simulink model "uloha3simulink"  (R2019b)
settings: Solver=FixedStepAuto  StartTime=0.0  StopTime=50  FixedStep=1e-3  MaxStep=1e-4  RelTol=1e-3
values from neighbouring files (symbols this model uses):
  B = 0.1    [uloha3.m]
  b = 0.05    [uloha3.m]
  Kd = G(3)    [uloha3.m]
  Ki = G(2)    [uloha3.m]
  Kp = G(1)    [uloha3.m]
  Kv = -1/g    (= -0.101936799185)    [uloha3.m]
  l = 3    [uloha3.m]
  omega = sqrt(g/l)    [uloha3.m]
  Tm = 1    [uloha3.m]
undefined symbols (not defined in the file or in its folder): A, jerk, Kd2, Ki2, Kp2, Nel, Tvz
libraries: simulink x3, vrlib x3
settings Model: Creator=Niki  LastModifiedBy=Niki

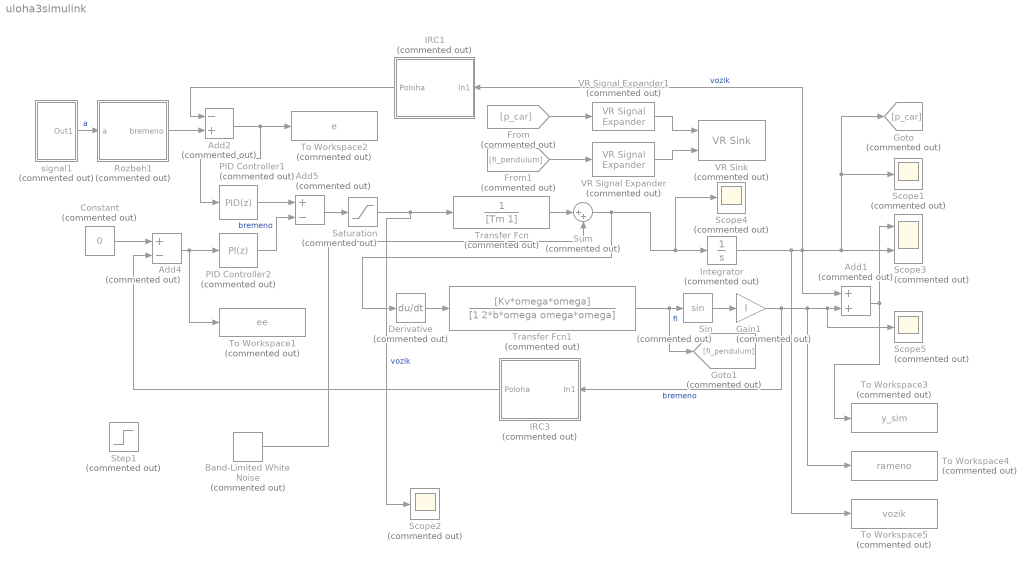
== system uloha3simulink ==
  Add1 : Sum  Commented=on
  Add2 : Sum  Commented=on  Inputs=-+
  Add4 : Sum  Commented=on  Inputs=+-
  Add5 : Sum  Commented=on  Inputs=+-
  Band-Limited White Noise : simulink/Sources/Band-Limited White Noise  Commented=on  Cov=[0.0005]  Ts=0.1  seed=[23341]
  Constant : Constant  Commented=on  Value=0
  Derivative : Derivative  Commented=on
  From : From  Commented=on  GotoTag=p_car
  From1 : From  Commented=on  GotoTag=fi_pendulum
  Gain1 : Gain  Commented=on  Gain=l
  Goto : Goto  Commented=on  GotoTag=p_car
  Goto1 : Goto  Commented=on  GotoTag=fi_pendulum
  IRC1 : Subsystem  Commented=on
  IRC3 : Subsystem  Commented=on
  Integrator : Integrator  Commented=on
  PID Controller1 : simulink/Continuous/PID Controller  Commented=on  Controller=PID  Form=Parallel  TimeDomain=Discrete-time  SampleTime=Tvz  IntegratorMethod=Forward Euler  FilterMethod=Forward Euler  ControllerParametersSource=internal  P=Kp  I=Ki  D=Kd  UseFilter=on  N=100  TunerSelectOption=Transfer Function Based (PID Tuner App)  InitialConditionSource=internal  InitialConditionForIntegrator=0  InitialConditionForFilter=0  DifferentiatorICPrevScaledInput=0  ExternalReset=none  TrackingMode=off  Kt=1  LimitOutput=off  UpperSaturationLimit=inf  LowerSaturationLimit=-inf  LinearizeAsGain=on  AntiWindupMode=none  Kb=1  POutMin=[]  POutMax=[]  IOutMin=[]  IOutMax=[]  DOutMin=[]  DOutMax=[]  NOutMin=[]  NOutMax=[]  SumOutMin=[]  SumOutMax=[]  SaturationOutMin=[]  SaturationOutMax=[]  PParamMin=[]  PParamMax=[]  IParamMin=[]  IParamMax=[]  DParamMin=[]  DParamMax=[]  NParamMin=[]  NParamMax=[]  KbParamMin=[]  KbParamMax=[]  KtParamMin=[]  KtParamMax=[]  KbOutMin=[]  KbOutMax=[]  KtOutMin=[]  KtOutMax=[]  IntegratorOutMin=[]  IntegratorOutMax=[]  FilterOutMin=[]  FilterOutMax=[]  SumI1OutMin=[]  SumI1OutMax=[]  SumI2OutMin=[]  SumI2OutMax=[]  SumI3OutMin=[]  SumI3OutMax=[]  SumI4OutMin=[]  SumI4OutMax=[]  SumDOutMin=[]  SumDOutMax=[]  DifferentiatorOutMin=[]  DifferentiatorOutMax=[]  FilterDiffOutCoefMin=[]  FilterDiffOutCoefMax=[]  ReciprocalOutMin=[]  ReciprocalOutMax=[]  SumDenOutMin=[]  SumDenOutMax=[]  SumNumOutMin=[]  SumNumOutMax=[]  DivideOutMin=[]  DivideOutMax=[]  IntegratorContinuousStateAttributes=''  IntegratorStateMustResolveToSignalObject=off  IntegratorRTWStateStorageClass=Auto  FilterContinuousStateAttributes=''  FilterStateMustResolveToSignalObject=off  FilterRTWStateStorageClass=Auto  ParallelPVariant=InternalParameters  IdealPVariant=Disabled  IVariant=InternalParameters  DVariant=InternalParameters  IntegratorVariant=Discrete  SatVariant=Disabled  AWVariant=Passthrough  PCopyVariant=Disabled  TRVariant=Disabled  FdbkBlocksVariant=Forward  IdealPFdbkVariant=Disabled  SatFdbkVariant=Disabled  DerivativeFilterVariant=ForwardEulerFilter  NVariant=InternalParameters  NCopyVariant=Disabled  FilterICVariant=InternalICsFilter  IntegratorICVariant=InternalICs  ExternalResetVariant=Disabled  TRSumVariant=Passthrough  SumFdbkVariant=Disabled  SumVariant=Sum_PID
  PID Controller2 : simulink/Continuous/PID Controller  Commented=on  Controller=PI  Form=Parallel  TimeDomain=Discrete-time  SampleTime=Tvz  IntegratorMethod=Forward Euler  FilterMethod=Forward Euler  ControllerParametersSource=internal  P=Kp2  I=Ki2  D=Kd2  UseFilter=on  N=100  TunerSelectOption=Transfer Function Based (PID Tuner App)  InitialConditionSource=internal  InitialConditionForIntegrator=0  InitialConditionForFilter=0  DifferentiatorICPrevScaledInput=0  ExternalReset=none  TrackingMode=off  Kt=1  LimitOutput=off  UpperSaturationLimit=inf  LowerSaturationLimit=-inf  LinearizeAsGain=on  AntiWindupMode=none  Kb=1  POutMin=[]  POutMax=[]  IOutMin=[]  IOutMax=[]  DOutMin=[]  DOutMax=[]  NOutMin=[]  NOutMax=[]  SumOutMin=[]  SumOutMax=[]  SaturationOutMin=[]  SaturationOutMax=[]  PParamMin=[]  PParamMax=[]  IParamMin=[]  IParamMax=[]  DParamMin=[]  DParamMax=[]  NParamMin=[]  NParamMax=[]  KbParamMin=[]  KbParamMax=[]  KtParamMin=[]  KtParamMax=[]  KbOutMin=[]  KbOutMax=[]  KtOutMin=[]  KtOutMax=[]  IntegratorOutMin=[]  IntegratorOutMax=[]  FilterOutMin=[]  FilterOutMax=[]  SumI1OutMin=[]  SumI1OutMax=[]  SumI2OutMin=[]  SumI2OutMax=[]  SumI3OutMin=[]  SumI3OutMax=[]  SumI4OutMin=[]  SumI4OutMax=[]  SumDOutMin=[]  SumDOutMax=[]  DifferentiatorOutMin=[]  DifferentiatorOutMax=[]  FilterDiffOutCoefMin=[]  FilterDiffOutCoefMax=[]  ReciprocalOutMin=[]  ReciprocalOutMax=[]  SumDenOutMin=[]  SumDenOutMax=[]  SumNumOutMin=[]  SumNumOutMax=[]  DivideOutMin=[]  DivideOutMax=[]  IntegratorContinuousStateAttributes=''  IntegratorStateMustResolveToSignalObject=off  IntegratorRTWStateStorageClass=Auto  FilterContinuousStateAttributes=''  FilterStateMustResolveToSignalObject=off  FilterRTWStateStorageClass=Auto  ParallelPVariant=InternalParameters  IdealPVariant=Disabled  IVariant=InternalParameters  DVariant=Disabled  IntegratorVariant=Discrete  SatVariant=Disabled  AWVariant=Passthrough  PCopyVariant=Disabled  TRVariant=Disabled  FdbkBlocksVariant=Forward  IdealPFdbkVariant=Disabled  SatFdbkVariant=Disabled  DerivativeFilterVariant=Disabled  NVariant=Disabled  NCopyVariant=Disabled_SignalSpec  FilterICVariant=Disabled  IntegratorICVariant=InternalICs  ExternalResetVariant=Disabled  TRSumVariant=Passthrough  SumFdbkVariant=Disabled  SumVariant=Sum_PI
  Rozbeh1 : Subsystem  Commented=on
  Saturation : Saturate  Commented=on  UpperLimit=5  LowerLimit=-5
  Scope{1..2,4..5} (4 alike) : Scope  Commented=on
  Scope3 : Scope  Commented=on  NumInputPorts=2
  Sin : Trigonometry  Commented=on
  Step1 : Step  Commented=on  Time=40  SampleTime=0
  Sum : Sum  Commented=on  Inputs=|++
  To Workspace1 : ToWorkspace  Commented=on  VariableName=ee  SampleTime=-1
  To Workspace2 : ToWorkspace  Commented=on  VariableName=e  SampleTime=-1
  To Workspace3 : ToWorkspace  Commented=on  VariableName=y_sim  SaveFormat=Timeseries  SampleTime=-1
  To Workspace4 : ToWorkspace  Commented=on  VariableName=rameno  SaveFormat=Timeseries  SampleTime=-1
  To Workspace5 : ToWorkspace  Commented=on  VariableName=vozik  SaveFormat=Timeseries  SampleTime=-1
  Transfer Fcn : TransferFcn  Commented=on  Denominator=[Tm 1]
  Transfer Fcn1 : TransferFcn  Commented=on  Numerator=[Kv*omega*omega]  Denominator=[1 2*b*omega omega*omega]
  VR Signal Expander : vrlib/VR Signal Expander  Commented=on  outwidth=4  outidx=[4]
      settings: SourceProductName=Simulink
  VR Signal Expander1 : vrlib/VR Signal Expander  Commented=on  outwidth=3  outidx=1
      settings: SourceProductName=Simulink
  VR Sink : vrlib/VR Sink  Commented=on  InstantiateOnLoad=on  SampleTime=0.1  ViewEnable=on  RemoteChange=off  RemoteView=off  FieldsWritten=Car.translation.3.1.1.double#klb.rotation.4.1.1.double  WorldFileName=vrml1.wrl  AutoView=off  VideoDimensions=[]  AllowVariableSize=off
      settings: SourceProductName=Simulink
  signal1 : Subsystem  Commented=on
  wires:
  Transfer Fcn1/1 -> Sin/1, Goto1/1  "fi"
  Sin/1 -> Gain1/1
  Integrator/1 -> IRC1/1(In1), Scope1/1, Goto/1, Scope3/2, Add1/1, To Workspace5/1  "vozik"
  Gain1/1 -> IRC3/1(In1), Scope5/1, Add1/2, To Workspace4/1  "bremeno"
  Add1/1 -> Scope3/1, To Workspace3/1
  Add4/1 -> To Workspace1/1, PID Controller2/1
  Constant/1 -> Add4/1
  PID Controller1/1 -> Add5/1
  Add5/1 -> Saturation/1
  Saturation/1 -> Scope2/1, Transfer Fcn/1  "vozik"
  Add2/1 -> To Workspace2/1, PID Controller1/1
  Rozbeh1/1(bremeno) -> Add2/2
  PID Controller2/1 -> Add5/2  "bremeno"
  VR Signal Expander/1 -> VR Sink/2
  VR Signal Expander1/1 -> VR Sink/1
  From/1 -> VR Signal Expander1/1
  From1/1 -> VR Signal Expander/1
  signal1/1(Out1) -> Rozbeh1/1(a)  "a"
  Derivative/1 -> Transfer Fcn1/1
  Transfer Fcn/1 -> Sum/1
  Sum/1 -> Derivative/1, Scope4/1, Integrator/1
  Band-Limited White Noise/1 -> Sum/2
  IRC3/1(Poloha) -> Add4/2
  IRC1/1(Poloha) -> Add2/1

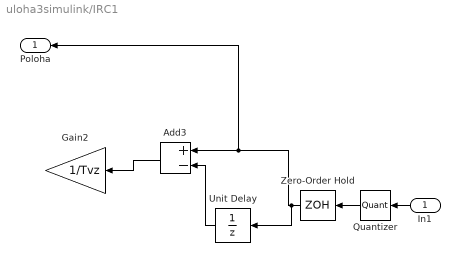
== system uloha3simulink/IRC1 ==
  In1 : Inport
  Add3 : Sum  Inputs=+-
  Gain2 : Gain  Gain=1/Tvz
  Quantizer : Quantizer  QuantizationInterval=2*pi/Nel
  Unit Delay : UnitDelay  SampleTime=Tvz  HasFrameUpgradeWarning=on
  Zero-Order Hold : ZeroOrderHold  SampleTime=Tvz
  Poloha : Outport
  wires:
  Quantizer/1 -> Zero-Order Hold/1
  In1/1 -> Quantizer/1
  Add3/1 -> Gain2/1
  Unit Delay/1 -> Add3/2
  Zero-Order Hold/1 -> Poloha/1, Add3/1, Unit Delay/1

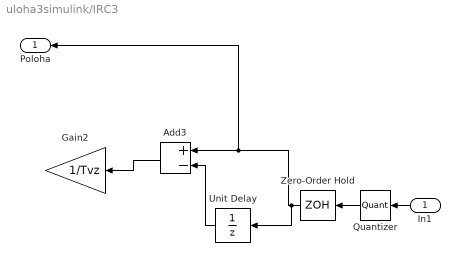
== system uloha3simulink/IRC3 ==
  In1 : Inport
  Add3 : Sum  Inputs=+-
  Gain2 : Gain  Gain=1/Tvz
  Quantizer : Quantizer  QuantizationInterval=2*pi/Nel
  Unit Delay : UnitDelay  SampleTime=Tvz  HasFrameUpgradeWarning=on
  Zero-Order Hold : ZeroOrderHold  SampleTime=Tvz
  Poloha : Outport
  wires:
  Zero-Order Hold/1 -> Unit Delay/1, Add3/1, Poloha/1
  Unit Delay/1 -> Add3/2
  Add3/1 -> Gain2/1
  In1/1 -> Quantizer/1
  Quantizer/1 -> Zero-Order Hold/1

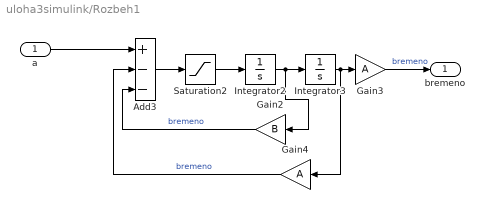
== system uloha3simulink/Rozbeh1 ==
  a : Inport
  Add3 : Sum  Inputs=+--
  Gain2 : Gain  Gain=B
  Gain3 : Gain  Gain=A
  Gain4 : Gain  Gain=A
  Integrator2 : Integrator
  Integrator3 : Integrator
  Saturation2 : Saturate  UpperLimit=jerk  LowerLimit=-jerk
  bremeno : Outport
  wires:
  a/1 -> Add3/1
  Saturation2/1 -> Integrator2/1
  Gain2/1 -> Add3/3  "bremeno"
  Add3/1 -> Saturation2/1
  Integrator3/1 -> Gain3/1, Gain4/1
  Gain4/1 -> Add3/2  "bremeno"
  Integrator2/1 -> Integrator3/1, Gain2/1
  Gain3/1 -> bremeno/1  "bremeno"

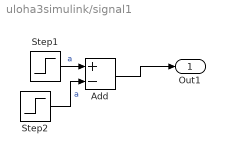
== system uloha3simulink/signal1 ==
  Add : Sum  Inputs=+-
  Step1 : Step  After=10  SampleTime=0
  Step2 : Step  Time=25  After=0  SampleTime=0
  Out1 : Outport
  wires:
  Add/1 -> Out1/1
  Step2/1 -> Add/2  "a"
  Step1/1 -> Add/1  "a"
